simulink model "MIPv2_hydro_LQR"  (R2015b)
settings: Solver=VariableStepAuto  StartTime=0.0  StopTime=tsim  RelTol=1e-3
undefined symbols (not defined in the file or in its folder): K, pinvTr, Ref, x_init
settings Model: Creator=Rotem  LastModifiedBy=Rotem

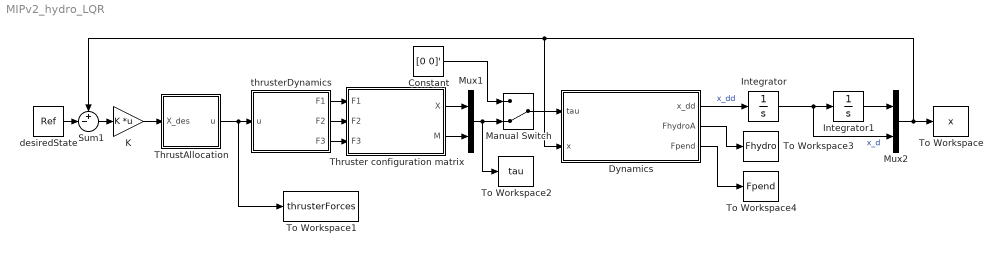
== system MIPv2_hydro_LQR ==
  Constant : Constant  Value=[0 0]'
  Dynamics : MATLAB Function  TreatAsAtomicUnit=on
  Integrator : Integrator  InitialCondition=x_init(4:6)
  Integrator1 : Integrator  InitialCondition=x_init(1:3)
  K : Gain  Gain=K  Multiplication=Matrix(K*u)
  Manual Switch : ManualSwitch  CurrentSetting=0
  Mux1 : Mux  Inputs=2
  Mux2 : Mux  Inputs=2
  Sum1 : Sum  Inputs=+-|
  ThrustAllocation : Subsystem
  Thruster configuration matrix : MATLAB Function  TreatAsAtomicUnit=on
  To Workspace : ToWorkspace  VariableName=x  SaveFormat=Timeseries  SampleTime=-1
  To Workspace1 : ToWorkspace  VariableName=thrusterForces  SaveFormat=Timeseries  SampleTime=-1
  To Workspace2 : ToWorkspace  VariableName=tau  SaveFormat=Timeseries  SampleTime=-1
  To Workspace3 : ToWorkspace  VariableName=Fhydro  SaveFormat=Timeseries  SampleTime=-1
  To Workspace4 : ToWorkspace  VariableName=Fpend  SaveFormat=Timeseries  SampleTime=-1
  desiredState : Constant  Value=Ref
  thrusterDynamics : Subsystem
  wires:
  Dynamics/1(x_dd) -> Integrator/1  "x_dd"
  Integrator/1 -> Mux2/2, Integrator1/1  "x_d"
  Thruster configuration matrix/1(X) -> Mux1/1
  Thruster configuration matrix/2(M) -> Mux1/2
  Constant/1 -> Manual Switch/1
  Mux1/1 -> To Workspace2/1, Manual Switch/2
  Manual Switch/1 -> Dynamics/1(tau)
  Integrator1/1 -> Mux2/1
  Dynamics/2(FhydroA) -> To Workspace3/1
  Dynamics/3(Fpend) -> To Workspace4/1
  desiredState/1 -> Sum1/2
  Sum1/1 -> K/1
  ThrustAllocation/1(u) -> To Workspace1/1, thrusterDynamics/1(u)
  K/1 -> ThrustAllocation/1(X_des)
  Mux2/1 -> Dynamics/2(x), Sum1/1, To Workspace/1
  thrusterDynamics/1(F1) -> Thruster configuration matrix/1(F1)
  thrusterDynamics/2(F2) -> Thruster configuration matrix/2(F2)
  thrusterDynamics/3(F3) -> Thruster configuration matrix/3(F3)

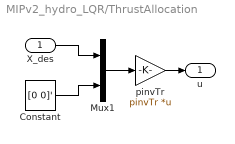
== system MIPv2_hydro_LQR/ThrustAllocation ==
  X_des : Inport
  Constant : Constant  Value=[0 0]'
  Mux1 : Mux  Inputs=2
  pinvTr : Gain  Gain=pinvTr  Multiplication=Matrix(K*u)
  u : Outport
  wires:
  pinvTr/1 -> u/1
  Constant/1 -> Mux1/2
  X_des/1 -> Mux1/1
  Mux1/1 -> pinvTr/1

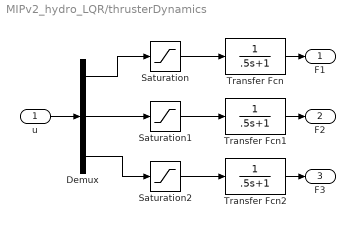
== system MIPv2_hydro_LQR/thrusterDynamics ==
  u : Inport
  Demux : Demux  Outputs=3
  Saturation : Saturate  UpperLimit=1.2  LowerLimit=-1.2
  Saturation1 : Saturate  UpperLimit=1.2  LowerLimit=-1.2
  Saturation2 : Saturate  UpperLimit=1.2  LowerLimit=-1.2
  Transfer Fcn : TransferFcn  Denominator=[.5 1]
  Transfer Fcn1 : TransferFcn  Denominator=[.5 1]
  Transfer Fcn2 : TransferFcn  Denominator=[.5 1]
  F1 : Outport
  F2 : Outport  Port=2
  F3 : Outport  Port=3
  wires:
  Transfer Fcn/1 -> F1/1
  Saturation/1 -> Transfer Fcn/1
  Transfer Fcn1/1 -> F2/1
  Saturation1/1 -> Transfer Fcn1/1
  Transfer Fcn2/1 -> F3/1
  Saturation2/1 -> Transfer Fcn2/1
  u/1 -> Demux/1
  Demux/1 -> Saturation/1
  Demux/2 -> Saturation1/1
  Demux/3 -> Saturation2/1

== matlab function MIPv2_hydro_LQR/Dynamics ==
  data: tau input; x input; x_dd output; FhydroA output; Fpend output
function [x_dd,FhydroA,Fpend]= MIPHdynamics(tau,x)

%% Input variables:
theta_0 = x(2);   theta_1 = x(3);
x_0d = x(4);  theta_0d = x(5);  theta_1d = x(6);
tau = [tau(1), tau(2), 0]';

%% Parameters:
g = 9.81;     % gravitational accleration
rho = 1000;   % [kg/m^3], density of water

% Vessel data:
m_0 = 6.34;   % [kg],     vessel mass
l_0 = 0.15;    % [m],      joint distance from center of pitch 
r = 0.548/2;  % [m],      radius of te CS Saucer
h = 0.129;    % [m]       total height of the CS Saucer
V = m_0/rho; % [m^3],    volume displacement = mass displacement/rho
I_y = (1/12)*m_0*(3*r^2+h^2); % [kgm^2], Mass moment of inertia about y axis
I_0 = I_y;
I_x = I_y;    % Cylindrical shape
% I_z = (m_0*r^2)/2; %[ kgm^2], mass moment of inertia about z axis
I_z = 0.116; %From Idland (2015)
I_g = diag([I_x I_y I_z]); % Inertia tensor
r_g = [0 0 0]'; % Location of CG wrt CO

% Pendulum data:
m_1 = 0.2;   % [kg],     pendulum mass
l_1 = 1.5;      % [m],      pendulum length 
I_1 = (m_1*(l_1)^2)/3; % [kg*m^2], pendulum inertia

% Added mass:
X_dotu = -3.50; %Added mass in surge due to surge motion
X_dotq = -0;    %Added mass in surge due to motion in pitch
M_dotu = -0;    %Added mass in pitch due to surge motion
M_dotq = -3;    %Added mass in pitch due to pitch motion

% Damping:
X_u = -1.96;    %Linear damping in surge due to surge motion
M_q = -3;       %Linear damping in pitch due to pitch motion
X_uu = -7.09;   %Nonlinear damping in surge due to surge motion
M_qq = -8;      %Nonlinear damping in pitch due to pitch motion

% Restoring:
I = (pi/4)*r^4; %[m^4], Area moment of inertia
KG = (.129/2);  %[m], KG for the Saucer. Assuming it is in the centre
KB  = 0.038/2;  %KB assuming it is in the centre of submerged volume
BM = I/V;       %BM_L = BM_T
BG = KG-KB;    
GM = BM-BG;     %GM (GM_L = GM_T)

%% System matrices with hydrodynamic coefficients:

% Hydroidynamic matrices
%Mass:
M_RB = [m_0*eye(3) -m_0*Smtrx(r_g);
        m_0*Smtrx(r_g) I_g];
M_A = -[X_dotu X_dotq;
        M_dotu M_dotq];
    
M = M_RB([1 5],[1 5]) + M_A; % 2 DOF mass     
M6 = zeros(6);      % Creating a 6 DOF mass matrix
M6([1 5],[1 5]) = M; %Inserting the relevant mass in the 6 by 6 matrix

%Restoring:
g_55 = rho*g*V*GM*sin(theta_0); % Fossen. p. 64

%Linear + nonlinear damping matrix, uncoupled motion:
Damp = -diag([X_u,M_q])-diag([X_uu*abs(x_0d),M_qq*abs(theta_0d)]); 

%Coriolis:
nu6=[x_0d 0 0 0 theta_0d 0]';
Cor6 = m2c(M6,nu6);     % Fossen p.180 
Cor = Cor6([1 5],[1 5]);  %Relevant Corliolis, surge and pitch

%3 "DOF" hydrodynamics:
M_A3 = zeros(3); M_A3(1:2,1:2) = M_A;
Rest3 = [0 g_55 0]';
Damp3 = zeros(3); Damp3(1:2,1:2) = Damp;
Cor3 = zeros(3); Cor3(1:2,1:2) = Cor;

%Pendulum dynamics: 
D_P = [m_0+m_1              m_1*l_0*cos(theta_0)             m_1*l_1*cos(theta_1)
     m_1*l_0*cos(theta_0) I_0+m_1*l_0^2                    m_1*l_0*l_1*cos(theta_0-theta_1)
     m_1*l_1*cos(theta_1) m_1*l_0*l_1*cos(theta_0-theta_1) m_1*l_1^2+I_1                   ];
C_P = [0 -m_1*l_0*sin(theta_0)*theta_0d             -m_1*l_1*sin(theta_1)*theta_1d
     0 0                                          m_1*l_0*l_1*sin(theta_0-theta_1)*theta_1d
     0 -m_1*l_0*l_1*sin(theta_0-theta_1)*theta_0d 0                                        ];
G_P = [0
     -m_1*g*l_0*sin(theta_0)
     -m_1*g*l_1*sin(theta_1)];

% % Assembling the matrices:
% D = [-X_dotu+m_0+m_1,     -X_dotq+m_1*l_0*cos(theta_0),    m_1*l_1*cos(theta_1);
%      -M_dotu+m_1*l_0*cos(theta_0),  -M_dotq+I_0+m_1*l_0^2,  m_1*l_0*l_1*cos(theta_0-theta_1);
%      m_1*l_1*cos(theta_1),   m_1*l_0*l_1*cos(theta_0-theta_1),     m_1*l_1^2+I_1          ];
%  
% C = [Cor(1,1)+Damp(1,1), Cor(1,2)+Damp(1,2)-m_1*l_0*sin(theta_0)*theta_0d, -m_1*l_1*sin(theta_1)*theta_1d;
%      Cor(2,1)+Damp(2,1),   Cor(2,2)+Damp(2,2),    m_1*l_0*l_1*sin(theta_0-theta_1)*theta_1d;
%      0,     -m_1*l_0*l_1*sin(theta_0-theta_1)*theta_0d,         0                         ];
%  
% G = [0
%      g_55-m_1*g*l_0*sin(theta_0)
%      -m_1*g*l_1*sin(theta_1)];



%% Solution:
% x_dd = D\(-C*x_d - G + tau);
Fhydro = +(Damp3*x(4:6)+Cor3*x(4:6)+Rest3); %Hydrodynamic forces
Fpend = +(C_P*x(4:6)+G_P); %"Pendulum" forces
x_dd = (D_P+M_A3)\(tau-Fhydro-Fpend); 
FhydroA = Fhydro+M_A3*x_dd; %Total hydrodynamic forces including added mass

== matlab function MIPv2_hydro_LQR/Thruster configuration matrix ==
  data: F1 input; X output; F2 input; F3 input; M output
function [X, M] = ThrustConfig(F1,F2,F3)
%Gives the forces and moments as output, input being the force from each
%motor.

rt = 0.135; %Radius from CG to motor axis in m
l_z = 0.1; %Moment arm in pitch (m)

u = [F1 F2 F3]'; %Control input (positive clockwise)

%Thrust configuration matrix, fixed azimuth angles (120 deg)
Tr=[0 sin(2*pi/3) sin(4*pi/3);1 cos(2*pi/3) cos(4*pi/3);rt rt rt];

tau = Tr*u; 

X = tau(1);
M = X*l_z; %Moment in pitch
